simulink model "measurements"  (R2022a)
settings: Solver=ode23tb  StartTime=0.0  StopTime=0.0015  MaxStep=1e-5  RelTol=1e-3
libraries: spsSeriesRLCBranchLib x8, spsGroundLib x5, spsVoltageMeasurementLib x4, spsVariableCapacitorLib x2, spsDiodeLib x2, spsControlledVoltageSourceLib x1, simulink_extras x1, eeGeneralControl x1, spsACVoltageSourceLib x1, spspowerguiLib x1
settings Model: Creator=stelt  LastModifiedBy=stelt

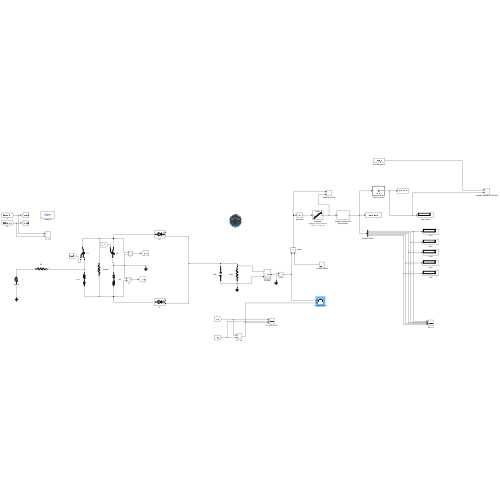
[thumbnail: Simulink's stored preview of the top-level diagram]
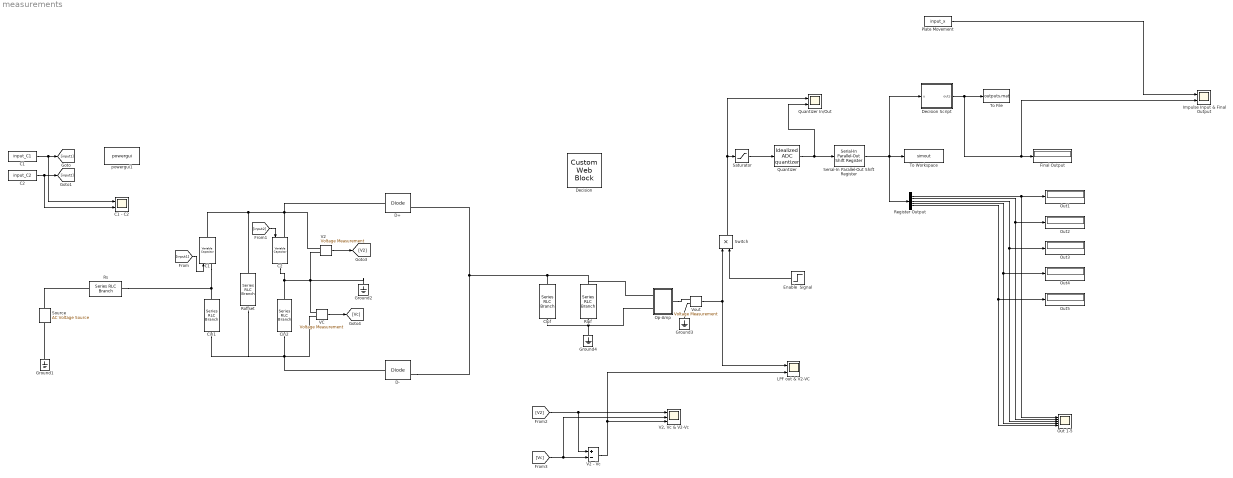
== system measurements ==
  C1 : spsVariableCapacitorLib/Variable Capacitor  methode=Backward Euler  Cabsmin=1e-10  Initialize=on  vC0=0  C0=4.43e-10  iC0=0
      settings: SourceProductBaseCode=PS
  "C1 " : FromWorkspace  VariableName=input_C1
  C1 - C2 : Scope  NumInputPorts=2
  C2 : spsVariableCapacitorLib/Variable Capacitor  methode=Backward Euler  Cabsmin=1e-10  Initialize=on  vC0=0  C0=4.43e-10  iC0=0
      settings: SourceProductBaseCode=PS
  "C2 " : FromWorkspace  VariableName=input_C2
  Cin1 : spsSeriesRLCBranchLib/Series RLC Branch  LConnTagsString=__new0  RConnTagsString=__new0  BranchType=RC  Resistance=1e-3  Inductance=0  SetiL0=off  InitialCurrent=0  Capacitance=4.43e-10  Setx0=off  InitialVoltage=0  Measurements=None
  Cin2 : spsSeriesRLCBranchLib/Series RLC Branch  LConnTagsString=__new0  RConnTagsString=__new0  BranchType=RC  Resistance=1e-3  Inductance=0  SetiL0=off  InitialCurrent=0  Capacitance=4.43e-10  Setx0=off  InitialVoltage=0  Measurements=None
  Clpf : spsSeriesRLCBranchLib/Series RLC Branch  LConnTagsString=__new0  RConnTagsString=__new0  BranchType=C  Resistance=1  Inductance=1e-3  SetiL0=off  InitialCurrent=0  Capacitance=1e-6  Setx0=off  InitialVoltage=0  Measurements=None
  D+ : spsDiodeLib/Diode  Ron=0.001  Lon=0  Vf=0.7  IC=0  UseSnubber=0  Rs=inf  Cs=0  Measurements=on
  D- : spsDiodeLib/Diode  Ron=0.001  Lon=0  Vf=0.7  IC=0  UseSnubber=0  Rs=inf  Cs=0  Measurements=on
  Decision : CustomWebBlock  LabelPosition=Hide  ShowInitialText=on  Configuration="{\"components\":[{\"name\":\"BackgroundImageComponent\",\"settings\":{\"image\":{\"size\":[150,150],\"src\":\"data:image\\/svg+xml;base64,PHN2ZyB4bWxucz0iaHR0cDovL3d3dy53My5vcmcvMjAwMC9zdmciIHhtbG5zOnhsaW5rPSJodHRwOi8vd3d3LnczLm9yZy8xOTk5L3hsaW5rIiB2aWV3Qm94PSIwIDAgNTAwIDUwMCI+PGRlZnM+PHN0eWxlPi5he2ZpbGw6dXJsKCNhKTt9LmJ7ZmlsbDp1cmwoI2IpO30uY3tmaWxsOnVybCgjYyk7fTwvc3R5bGU+PHJhZGlhbEdyYWRpZW50IGlkPSJhIiBjeD0iMjgzLjg0IiBjeT0iLTQ2Ni4zNyIgcj0iMzc1Ljc1IiBncmFkaWVudFRyYW5zZm9ybT0ibWF0cml4KDEuMzksIDAsIDAsIC0xLjM5LCAtMTUzLjU2LCAtNjQ0LjA4KSIg ...(+2088 chars)\",\"srcOrientation\":\"Right\"},\"position\":[0,0,1,1],\"scaleMode\":\"0\"}},{\"name\":\"LampStateComponent\",\"settings\":{\"position\":[0,0,1,1],\"states\":[{\"icon\":{\"customSrc\":\"data:image\\/svg+xml;base64,PHN2ZyBpZD0iTGF5ZXJfMSIgZGF0YS1uYW1lPSJMYXllciAxIiB4bWxucz0iaHR0cDovL3d3dy53My5vcmcvMjAwMC9zdmciIHZpZXdCb3g9IjAgMCA0MTEgNDU4Ij48ZGVmcz48c3R5bGU+LmNscy0xe2ZpbGw6I2ZkZjhjMTt9LmNscy0ye2ZpbGw6I2ZlZTEwMDt9LmNscy0ze2ZpbGw6IzIzMWYyMDt9LmNscy00e2ZpbGw6I2EwOWY5Zjt9LmNscy00LC5jbHMtNSwuY2xzLTZ7c3Ryb2tlOiMyMzFmMjA7c3Ryb2tlLW1pdGVybGltaXQ6MTA7fS5jbHMtNXtmaWxsOiNmZmY7fS5jbHMtNntmaWxsOm5vbmU7fTwvc3R5bGU+PC9kZWZz ...(+5168 chars)\",\"id\":-1,\"srcOrientation\":\"Right\",\"type\":\"custom\"},\"iconScale\":0.8,\"metadata\":{},\"overlayType\":\"intersect\",\"shape\":{\"color\":[0.725,0,0],\"opacity\":1,\"position\":[0.1,0.1,0.8,0.8],\"type\":\"ellipse\"},\"value\":null},{\"icon\":{\"customSrc\":\"data:image\\/svg+xml;base64,PHN2ZyBpZD0iTGF5ZXJfMSIgZGF0YS1uYW1lPSJMYXllciAxIiB4bWxucz0iaHR0cDovL3d3dy53My5vcmcvMjAwMC9zdmciIHZpZXdCb3g9IjAgMCA0MTEgNDU4Ij48ZGVmcz48c3R5bGU+LmNscy0xe2ZpbGw6I2ZkZjhjMTt9LmNscy0ye2ZpbGw6I2ZlZTEwMDt9LmNscy0ze2ZpbGw6IzIzMWYyMDt9LmNscy00e2ZpbGw6I2EwOWY5Zjt9LmNscy00LC5jbHMtNSwuY2xzLTZ7c3Ryb2tlOiMyMzFmMjA7c3Ryb2tlLW1pdGVybGltaXQ6MTA7fS5jbHMtNXtmaWxsOiNmZmY7fS5jbHMtNntmaWxsOm5vbmU7fTwvc3R5bGU+PC9kZWZz ...(+5168 chars)\",\"id\":-1,\"srcOrientation\":\"Right\",\"type\":\"custom\"},\"iconScale\":0.8,\"metadata\":{\"useDefaults\":{\"customIcon\":true,\"icon\":true,\"overlayType\":true,\"shape\":true,\"sizeAndPosition\":true}},\"overlayType\":\"intersect\",\"shape\":{\"color\":[0,0,0],\"opacity\":1,\"position\":[0.1,0.1,0.8,0.8],\"type\":\"ellipse\"},\"value\":\"0\"},{\"icon\":{\"customSrc\":\"data:image\\/svg+xml;base64,PHN2ZyBpZD0iTGF5ZXJfMSIgZGF0YS1uYW1lPSJMYXllciAxIiB4bWxucz0iaHR0cDovL3d3dy53My5vcmcvMjAwMC9zdmciIHZpZXdCb3g9IjAgMCA0MTEgNDU4Ij48ZGVmcz48c3R5bGU+LmNscy0xe2ZpbGw6I2ZkZjhjMTt9LmNscy0ye2ZpbGw6I2ZlZTEwMDt9LmNscy0ze2ZpbGw6IzIzMWYyMDt9LmNscy00e2ZpbGw6I2EwOWY5Zjt9LmNscy00LC5jbHMtNSwuY2xzLTZ7c3Ryb2tlOiMyMzFmMjA7c3Ryb2tlLW1pdGVybGltaXQ6MTA7fS5jbHMtNXtmaWxsOiNmZmY7fS5jbHMtNntmaWxsOm5vbmU7fTwvc3R5bGU+PC9kZWZz ...(+5168 chars)\",\"id\":-1,\"srcOrientation\":\"Right\",\"type\":\"custom\"},\"iconScale\":0.8,\"metadata\":{\"useDefaults\":{\"customIcon\":true,\"icon\":true,\"overlayType\":true,\"shape\":true,\"sizeAndPosition\":true}},\"overlayType\":\"intersect\",\"shape\":{\"color\":[0.988,0.988,0.773],\"opacity\":1,\"position\":[0.1,0.1,0.8,0.8],\"type\":\"ellipse\"},\"value\":\"1\"}],\"valueType\":\"discrete\"}},{\"name\":\"ForegroundImageComponent\",\"settings\":{\"image\":{\"size\":[150,150],\"src\":\"data:image\\/svg+xml;base64,PHN2ZyB4bWxucz0iaHR0cDovL3d3dy53My5vcmcvMjAwMC9zdmciIHhtbG5zOnhsaW5rPSJodHRwOi8vd3d3LnczLm9yZy8xOTk5L3hsaW5rIiB2aWV3Qm94PSIwIDAgNTAwIDUwMCI+PGRlZnM+PHN0eWxlPi5he2ZpbGw6dXJsKCNhKTt9PC9zdHlsZT48bGluZWFyR3JhZGllbnQgaWQ9ImEiIHgxPSIxNzMuMDUiIHkxPSItNjI3Ljc4IiB4Mj0iMTczLjA1IiB5Mj0iLTUyMi40MyIgZ3JhZGllbnRUcmFuc2Zvcm09Im1hdHJpeCgxLjI5LCAwLCAwLCAtMS4zMywgMjcuMTMsIC02MjguMzEpIiBncmFkaWVudFVuaXRzPSJ1c2VyU3BhY2VPblVzZSI+PHN0b3Agb2Zmc2V0PSIwIiBzdG9wLWNvbG9yPSIjZmZmIiBzdG9wLW9wYWNpdHk9IjAuMjUiLz48c3RvcCBvZmZzZXQ9IjEiIHN0b3AtY29sb3I9IiNmZmYiIHN0b3Atb3BhY2l0eT0iMCIvPjwvbGluZWFyR3JhZGllbnQ+PC9kZWZzPjxwYXRoIGNsYXNzPSJhIiBkPSJNNDI5LjMsMTkwLjY2QzQwMi40NSwxMTQuNTEsMzMyLjY3LDYwLjE3LDI1MC44NSw2MC4xN2MtODMuNDMsMC0xNTQuMjgsNTYuNDItMTc5Ljk1LDEzNSwxNS4zNCwzOSw4OC4xMSw3LDE3Ny4wNyw3QzM0MCwyMDIuMDgsNDE3LjI2LDIzNi40Niw0MjkuMywxOTAuNjZaIi8+PC9zdmc+\",\"srcOrientation\":\"Right\"},\"isForeground\":1,\"position\":[0,0,1,1],\"scaleMode\":\"0\"}}],\"settings\":{\"BindingType\":\"signal\",\"aspectRatio\":1.032258064516129,\"backgroundColor\":[0,0,0],\"backgroundOffset\":0.14,\"backgroundOpacity\":1,\"blockOrientation\":\"Right\",\"fixedAspectRatio\":\"on\",\"showBackgroundColor\":false,\"value\":0,\"version\":\"22a\"},\"type\":\"Lamp\"}"
  Decision Script : MATLAB Function  TreatAsAtomicUnit=on
  Enable  Signal : Step  Time=3e-4  SampleTime=0
  Final Output : Display
  Ground{1..4} (4 alike) : spsGroundLib/Ground  LConnTagsString=a
  Impulse Input & Final Output : Scope  NumInputPorts=2
  LPF out & V2-VC : Scope  NumInputPorts=2
  Op-Amp : Subsystem
  Out 1-5 : Scope  NumInputPorts=5
  Out{1..5} (5 alike) : Display
  Plate Movement : FromWorkspace  VariableName=input_x
  Quantizer : simulink_extras/Additional Discrete/Idealized ADC quantizer  NumberOfConverterBits=8  Vmin=0  Vmax=4  OutputDataType=uint8  OutputNegativeValues=off
  Quantizer In/Out : Scope  NumInputPorts=2
  Register Output : Demux  Outputs=5
  Rlpf : spsSeriesRLCBranchLib/Series RLC Branch  LConnTagsString=__new0  RConnTagsString=__new0  BranchType=R  Resistance=100  Inductance=1e-3  SetiL0=off  InitialCurrent=0  Capacitance=1e-6  Setx0=off  InitialVoltage=0  Measurements=None
  Roffset : spsSeriesRLCBranchLib/Series RLC Branch  LConnTagsString=__new0  RConnTagsString=__new0  BranchType=R  Resistance=1e6  Inductance=0  SetiL0=off  InitialCurrent=0  Capacitance=0  Setx0=off  InitialVoltage=0  Measurements=None
  Rs : spsSeriesRLCBranchLib/Series RLC Branch  LConnTagsString=__new0  RConnTagsString=__new0  BranchType=R  Resistance=0.1  Inductance=0  SetiL0=off  InitialCurrent=0  Capacitance=0  Setx0=off  InitialVoltage=0  Measurements=None
  Saturator : Saturate  UpperLimit=4  LowerLimit=0
  Serial-In Parallel-Out Shift Register : eeGeneralControl/Serial-In Parallel-Out Shift Register  N=5  IC=0  Ts=1e-6
      settings: SourceProductBaseCode=PS
  Source : spsACVoltageSourceLib/AC Voltage Source  Amplitude=12  Phase=0  Frequency=1e4  SampleTime=0  Measurements=None  BusType=swing  Pref=10e3  Qref=0  Qmin=-inf  Qmax=+inf
  Switch : Product  Inputs=**
  To File : ToFile  Filename=outputs.mat  MatrixName=outputs
  To Workspace : ToWorkspace  VariableName=simout  SaveFormat=Timeseries  SampleTime=-1
  V2 : spsVoltageMeasurementLib/Voltage Measurement  PhasorSimulation=off  OutputType=Complex  PSBequivalent=0
  V2 - Vc : Sum  Inputs=+-
  "V2, Vc & V2-Vc" : Scope  NumInputPorts=3
  VC : spsVoltageMeasurementLib/Voltage Measurement  PhasorSimulation=off  OutputType=Complex  PSBequivalent=0
  Vout : spsVoltageMeasurementLib/Voltage Measurement  PhasorSimulation=off  OutputType=Complex  PSBequivalent=0
  powergui1 : spspowerguiLib/powergui  Priority=1  SimulationMode=Discrete  SampleTime=1e-7  frequency=60  Iterations=50  frequencyindice=0  Pbase=100e6  ErrMax=1e-4  UnitsV=kV  UnitsW=MW  buscounter=0  FunctionMessages=off  echomessages=off  EnableUseOfTLC=off  CurrentSourceSwitches=off  DisableSnubberDevices=off  DisableRonSwitches=off  DisableVfSwitches=off  DisplayEquations=off  AutomaticDiscreteSolvers=off  SolverType=Tustin/Backward Euler (TBE)  Interpol=off  ExternalGateDelay=off  methode=off  Ts=100  x0status=blocks  SPID=on  SwTol=0  HookPort=off  NonlinearTolerance=1e-4  nMaxIteration=100  ContinueOnMaxIteration=off  RestoreLinks=warning  ResistiveCurrentMeasurement=off  Frange=[0:2:500]  Ylog=off  Xlog=on  ShowGrid=off  save=off  variable=ZData  structure=0  ZoomFFT=off  StartTime=0.0  cycles=1  DisplayStyle=1  fundamental=60  FreqAxis=off  MaxFrequency=1000  frequencyindicesteady=1  RmsSteady=1  display=off
  wires:
  [input1] -> C1/1
  [V2] -> V2 - Vc/1, "V2, Vc & V2-Vc"/1
  V2/1 -> [V2]
  [input2] -> C2/1
  VC/1 -> [Vc]
  V2 - Vc/1 -> "V2, Vc & V2-Vc"/3, LPF out & V2-VC/2
  "C1 "/1 -> C1 - C2/1, [input1]
  "C2 "/1 -> C1 - C2/2, [input2]
  [Vc] -> "V2, Vc & V2-Vc"/2, V2 - Vc/2
  Vout/1 -> Switch/1, LPF out & V2-VC/1
  Saturator/1 -> Quantizer/1
  Serial-In Parallel-Out Shift Register/1 -> Register Output/1, To Workspace/1, Decision Script/1(u)
  Decision Script/1(outs) -> Impulse Input & Final Output/2, Final Output/1, To File/1
  Quantizer/1 -> Quantizer In/Out/2, Serial-In Parallel-Out Shift Register/1
  Register Output/1 -> Out 1-5/1, Out1/1
  Register Output/2 -> Out 1-5/2, Out2/1
  Register Output/3 -> Out 1-5/3, Out3/1
  Switch/1 -> Quantizer In/Out/1, Saturator/1
  Enable  Signal/1 -> Switch/2
  Register Output/5 -> Out 1-5/5, Out5/1
  Register Output/4 -> Out 1-5/4, Out4/1
  Plate Movement/1 -> Impulse Input & Final Output/1
  connections:
  Cin2/LConn1 -- Roffset/RConn1 -- Cin1/RConn1 -- D-/LConn1 -- VC/LConn1
  C1/LConn1 -- Rs/RConn1 -- Cin1/LConn1
  Ground1/LConn1 -- Source/LConn1
  Rs/LConn1 -- Source/RConn1
  D-/RConn1 -- Op-Amp/LConn1 -- Rlpf/LConn1 -- Clpf/LConn1 -- D+/RConn1
  Rlpf/RConn1 -- Clpf/RConn1 -- Op-Amp/LConn2 -- Ground4/LConn1
  Op-Amp/RConn1 -- Vout/LConn1
  Ground3/LConn1 -- Vout/LConn2
  D+/LConn1 -- V2/LConn1 -- C2/LConn1 -- Roffset/LConn1 -- C1/RConn1
  VC/LConn2 -- V2/LConn2 -- Ground2/LConn1 -- C2/RConn1 -- Cin2/RConn1

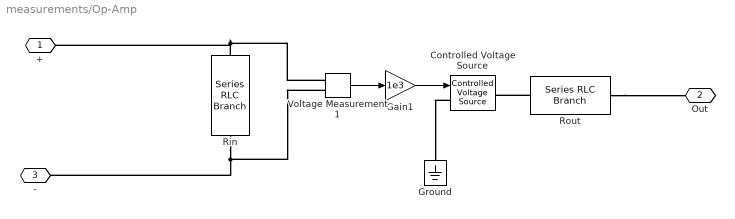
== system measurements/Op-Amp ==
  Controlled Voltage Source : spsControlledVoltageSourceLib/Controlled Voltage Source  Initialize=on  Source_Type=DC  Amplitude=0  Phase=0  Frequency=0  Measurements=None
  Gain1 : Gain  Gain=1e3
  Ground : spsGroundLib/Ground  LConnTagsString=a
  Rin : spsSeriesRLCBranchLib/Series RLC Branch  LConnTagsString=__new0  RConnTagsString=__new0  BranchType=R  Resistance=1e12  Inductance=1e-3  SetiL0=off  InitialCurrent=0  Capacitance=1e-6  Setx0=off  InitialVoltage=0  Measurements=None
  Rout : spsSeriesRLCBranchLib/Series RLC Branch  LConnTagsString=__new0  RConnTagsString=__new0  BranchType=R  Resistance=0.001  Inductance=1e-3  SetiL0=off  InitialCurrent=0  Capacitance=1e-6  Setx0=off  InitialVoltage=0  Measurements=None
  Voltage Measurement1 : spsVoltageMeasurementLib/Voltage Measurement  PhasorSimulation=off  OutputType=Complex  PSBequivalent=0
  + : PMIOPort  Side=Left
  Out : PMIOPort  Port=2  Side=Right
  - : PMIOPort  Port=3  Side=Left
  wires:
  Voltage Measurement1/1 -> Gain1/1
  Gain1/1 -> Controlled Voltage Source/1
  connections:
  Rin/RConn1 -- Voltage Measurement1/LConn2 -- -/RConn1
  Rout/RConn1 -- Out/RConn1
  Controlled Voltage Source/LConn1 -- Ground/LConn1
  Rin/LConn1 -- Voltage Measurement1/LConn1 -- +/RConn1
  Rout/LConn1 -- Controlled Voltage Source/RConn1

== matlab function measurements/Decision Script ==
  data: u input; outs output
function outs = fcn(u)

threshold = 180;

y = 0;
if (u(1)+u(2)+u(3)+u(4)+u(5))/5 > threshold
y = 1;
end

outs = y;
